simulink model "LABORATORY2"  (R2023b)
settings: Solver=VariableStepAuto  StartTime=0.0  StopTime=10.0  RelTol=1e-3
values from neighbouring files (symbols this model uses):
  G1_den = [1 2 1]    [LABORATORY2.m]    (also in LABORATORY2_Code.m)
  G1_num = [1]    [LABORATORY2.m]    (also in LABORATORY2_Code.m)
  G2_den = conv(G2_denA,G2_denB)    [LABORATORY2.m]    (also in LABORATORY2_Code.m)
  G2_num = [1]    [LABORATORY2.m]    (also in LABORATORY2_Code.m)
  G3_den = conv(G3_denA,G3_denB)    [LABORATORY2.m]    (also in LABORATORY2_Code.m)
  G3_num = [1]    [LABORATORY2.m]    (also in LABORATORY2_Code.m)
  G4_den = [1 1]    [LABORATORY2.m]    (also in LABORATORY2_Code.m)
  G4_num = [1]    [LABORATORY2.m]    (also in LABORATORY2_Code.m)
  G5_den = [1 2 3 4 5 6 7 1]    [LABORATORY2.m]    (also in LABORATORY2_Code.m)
  G5_num = [8 7 6 5 4 3 2]    [LABORATORY2.m]    (also in LABORATORY2_Code.m)
  G6_den = [1 2 3 4 1]    [LABORATORY2.m]    (also in LABORATORY2_Code.m)
  G6_num = [4 3 2 1]    [LABORATORY2.m]    (also in LABORATORY2_Code.m)
  G7_den = [1 2 3 4 5 1]    [LABORATORY2.m]    (also in LABORATORY2_Code.m)
  G7_num = [6 5 4 3 2]    [LABORATORY2.m]    (also in LABORATORY2_Code.m)
  G8_den = [1 3 5 7 9 1]    [LABORATORY2.m]    (also in LABORATORY2_Code.m)
  G8_num = [10 8 6 4 2]    [LABORATORY2.m]    (also in LABORATORY2_Code.m)
settings Model: Creator=USER  LastModifiedBy=USER

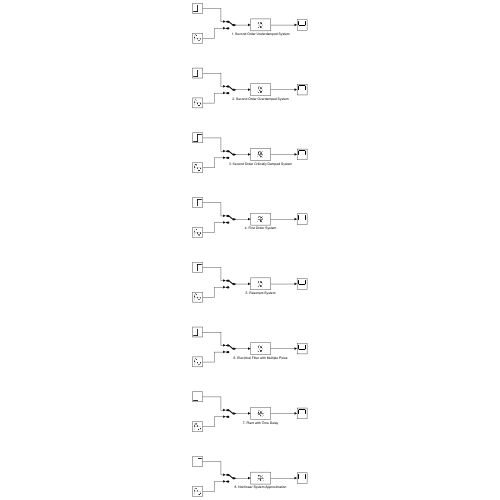
[thumbnail: Simulink's stored preview of the top-level diagram]
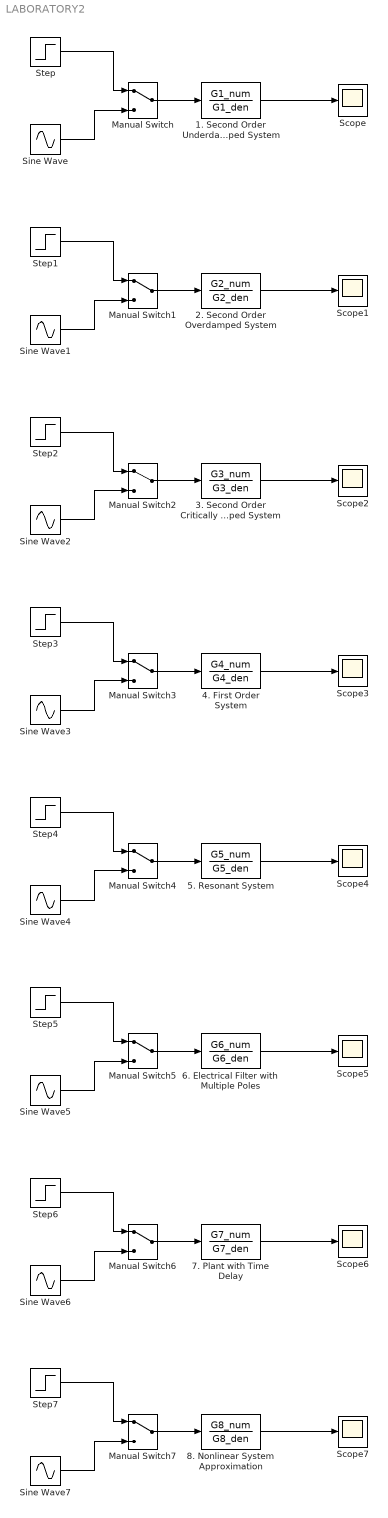
== system LABORATORY2 ==
  1. Second Order Underdamped System : TransferFcn  Numerator=G1_num  Denominator=G1_den
  2. Second Order Overdamped System : TransferFcn  Numerator=G2_num  Denominator=G2_den
  3. Second Order Critically Damped System : TransferFcn  Numerator=G3_num  Denominator=G3_den
  4. First Order System : TransferFcn  Numerator=G4_num  Denominator=G4_den
  5. Resonant System : TransferFcn  Numerator=G5_num  Denominator=G5_den
  6. Electrical Filter with Multiple Poles : TransferFcn  Numerator=G6_num  Denominator=G6_den
  7. Plant with Time Delay : TransferFcn  Numerator=G7_num  Denominator=G7_den
  8. Nonlinear System Approximation : TransferFcn  Numerator=G8_num  Denominator=G8_den
  Manual Switch{,1..7} (8 alike) : ManualSwitch
  Scope{,1..7} (8 alike) : Scope
  Sine Wave{,1..7} (8 alike) : Sin  SampleTime=0
  Step{,1..7} (8 alike) : Step  SampleTime=0
  wires:
  Step/1 -> Manual Switch/1
  Sine Wave/1 -> Manual Switch/2
  Manual Switch/1 -> 1. Second Order Underdamped System/1
  1. Second Order Underdamped System/1 -> Scope/1
  Sine Wave1/1 -> Manual Switch1/2
  Step1/1 -> Manual Switch1/1
  Manual Switch1/1 -> 2. Second Order Overdamped System/1
  2. Second Order Overdamped System/1 -> Scope1/1
  3. Second Order Critically Damped System/1 -> Scope2/1
  Step2/1 -> Manual Switch2/1
  Sine Wave2/1 -> Manual Switch2/2
  Manual Switch2/1 -> 3. Second Order Critically Damped System/1
  Manual Switch3/1 -> 4. First Order System/1
  4. First Order System/1 -> Scope3/1
  Step3/1 -> Manual Switch3/1
  Sine Wave3/1 -> Manual Switch3/2
  Sine Wave4/1 -> Manual Switch4/2
  5. Resonant System/1 -> Scope4/1
  Step4/1 -> Manual Switch4/1
  Manual Switch4/1 -> 5. Resonant System/1
  Manual Switch5/1 -> 6. Electrical Filter with Multiple Poles/1
  6. Electrical Filter with Multiple Poles/1 -> Scope5/1
  Step5/1 -> Manual Switch5/1
  Sine Wave5/1 -> Manual Switch5/2
  Manual Switch6/1 -> 7. Plant with Time Delay/1
  Sine Wave6/1 -> Manual Switch6/2
  Step6/1 -> Manual Switch6/1
  7. Plant with Time Delay/1 -> Scope6/1
  Step7/1 -> Manual Switch7/1
  Sine Wave7/1 -> Manual Switch7/2
  8. Nonlinear System Approximation/1 -> Scope7/1
  Manual Switch7/1 -> 8. Nonlinear System Approximation/1
